simulink model "simulation_ex_2_2014a"  (R2014a)
settings: Solver=ode45  SolverMode=SingleTasking  StartTime=0.0  StopTime=250  RelTol=1e-3
settings Model: CovMetricSettings=dwe  CovHtmlReporting=off  covSaveCumulativeToWorkspaceVar=off  CovSaveSingleToWorkspaceVar=off  CovExternalEMLEnable=on  CovSFcnEnable=on  Creator=HanO  LastModifiedBy=HanO
settings DataIOCC: LimitDataPoints=off  SaveFormat=StructureWithTime  ReturnWorkspaceOutputs=on
settings DebuggingCC: MergeDetectMultiDrivingBlocksExec=error  SolverPrmCheckMsg=none  FrameProcessingCompatibilityMsg=error  SFUnexpectedBacktrackingDiag=error  SFNoUnconditionalDefaultTransitionDiag=error
settings HardwareCC: ProdBitPerPointer=64  ProdLargestAtomicFloat=Float  ProdIntDivRoundTo=Zero  ProdEndianess=LittleEndian  ProdHWDeviceType=Specified
settings ModelReferenceCC: PropagateSignalLabelsOutOfModel=on
settings SFSimCC: SimUseLocalCustomCode=on
settings RTWCC: RTWUseLocalCustomCode=on
settings GRTTargetCC: TargetLangStandard=C99 (ISO)

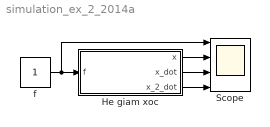
== system simulation_ex_2_2014a ==
  He giam xoc : Subsystem  mask{k=0.2, b=0.1, m=2, x0=0.1}
      mask prompts: k "Độ cứng lò xo k ="; b "Hệ số ma sát nhớt b ="; m "Khối lượng vật nặng m ="; x0 "Vị trí ban đầu x0 ="
  Scope : Scope  NumInputPorts=4
      settings: TimeRange=auto  MaxDataPoints=5000  SaveName=ScopeData  YMin=0.9~-0.98284~-1.36372~-0.49623  YMax=1.1~9.84552~1.62622~0.59958  SampleTime=-1
  f : Constant
  wires:
  f/1 -> Scope/1, He giam xoc/1(f)
  He giam xoc/3(x_2_dot) -> Scope/4
  He giam xoc/2(x_dot) -> Scope/3
  He giam xoc/1(x) -> Scope/2

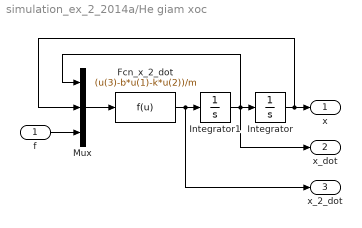
== system simulation_ex_2_2014a/He giam xoc ==
  f : Inport
  Fcn_x_2_dot : Fcn  Expr=(u(3)-b*u(1)-k*u(2))/m
  Integrator : Integrator  InitialCondition=x0
  Integrator1 : Integrator
  Mux : Mux  Inputs=3
  x : Outport
  x_dot : Outport  Port=2
  x_2_dot : Outport  Port=3
  wires:
  Fcn_x_2_dot/1 -> x_2_dot/1, Integrator1/1
  Mux/1 -> Fcn_x_2_dot/1
  f/1 -> Mux/3
  Integrator1/1 -> Mux/1, x_dot/1, Integrator/1
  Integrator/1 -> Mux/2, x/1
